simulink model "chap2_4sim"  (Simulink 7.7)
settings: Solver=ode45  SolverMode=SingleTasking  StartTime=0.0  StopTime=20  FixedStep=0.00001  RelTol=1e-3  AbsTol=1e-3
settings Model: Creator=liujk  LastModifiedBy=ljk  ExtModeTrigMode=oneshot  ExtModeArmWhenConnect=off
settings DataIOCC: LimitDataPoints=off
settings OptimizationCC: BlockReduction=off  BooleanDataType=off  ExpressionDepthLimit=128
settings DebuggingCC: SaveWithParameterizedLinksMsg=none  SignalResolutionControl=TryResolveAllWithWarning  SolverPrmCheckMsg=none  MultiTaskDSMMsg=warning  MultiTaskCondExecSysMsg=none  FcnCallInpInsideContextMsg=Enable All  StrictBusMsg=None
settings HardwareCC: TargetUnknown=on
settings RTWCC: IncludeERTFirstTime=on
settings CodeAppCC: CustomSymbolStrType=$N$R$M_T

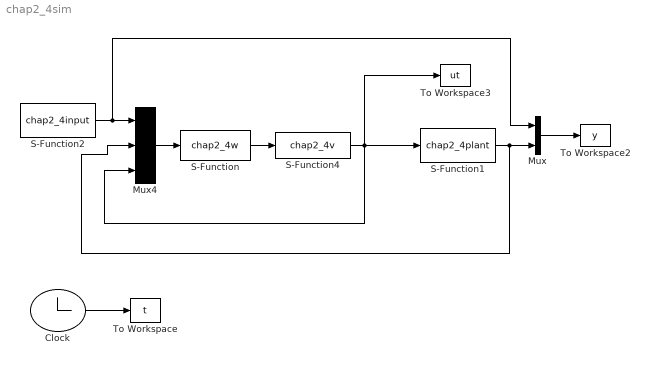
== system chap2_4sim ==
  Clock : Clock
  Mux : Mux  Inputs=2
  Mux4 : Mux  Inputs=3
  S-Function : S-Function  FunctionName=chap2_4w  EnableBusSupport=off
  S-Function1 : S-Function  FunctionName=chap2_4plant  EnableBusSupport=off
  S-Function2 : S-Function  FunctionName=chap2_4input  EnableBusSupport=off
  S-Function4 : S-Function  FunctionName=chap2_4v  EnableBusSupport=off
  To Workspace : ToWorkspace  VariableName=t  SampleTime=-1  SaveFormat=Array
  To Workspace2 : ToWorkspace  VariableName=y  SampleTime=-1  SaveFormat=Array
  To Workspace3 : ToWorkspace  VariableName=ut  SampleTime=-1  SaveFormat=Array
  wires:
  Mux4/1 -> S-Function/1
  Mux/1 -> To Workspace2/1
  S-Function1/1 -> Mux/2, Mux4/2
  S-Function2/1 -> Mux4/1, Mux/1
  Clock/1 -> To Workspace/1
  S-Function/1 -> S-Function4/1
  S-Function4/1 -> Mux4/3, To Workspace3/1, S-Function1/1
